simulink model "chap2_6sim"  (Simulink 6.3)
settings: Solver=ode45  StartTime=0.0  StopTime=10  RelTol=1e-3
values from neighbouring files (symbols this model uses):
  K = 1    [chap2_3.m]    (also in chap2_6int.m = 10; chap2_7.m = Kp*tf([1 wi],[1 0]))
  tol = 80    [chap2_3.m]    (also in chap2_6int.m = 1; chap2_9.m)
settings Model: LastModifiedBy=Administrator  ExtModeTrigMode=oneshot  ExtModeArmWhenConnect=off  StrictBusMsg=None
settings DataIOCC: LimitDataPoints=off  SignalLoggingName=sigsOut
settings OptimizationCC: BooleanDataType=off
settings DebuggingCC: SolverPrmCheckMsg=none
settings HardwareCC: TargetUnknown=on

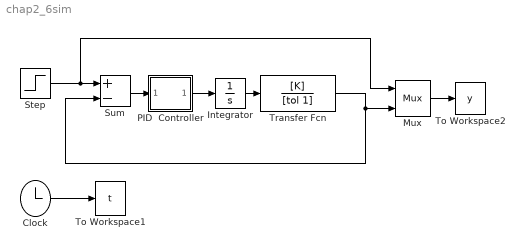
== system chap2_6sim ==
  Clock : Clock
      settings: Decimation=10
  Integrator : Integrator
  Mux : Mux  Inputs=2
  PID  Controller : Subsystem  mask(PID Controller){@1=Kp, @2=0, @3=Kd}
      mask prompts: @1 "Proportional:"; @2 "Integral"; @3 "Derivative:"
      mask help:
      | Enter expressions for proportional, integral, and derivative terms.
      | P+I/s+Ds
      mask init:
      | P=@1; I=@2; D=@3;
      mask Help: This block implements a PID controller where parameters are entered for the Proportional, Integral and Derivative terms. Unmask this block to see how it works. The derivative term is implemented using a true derivative block.
      mask Display: disp('PID')
  Step : Step  Time=0  SampleTime=0
  Sum : Sum  Inputs=+-  SaturateOnIntegerOverflow=on  InputSameDT=on
  To Workspace1 : ToWorkspace  VariableName=t  SampleTime=-1  SaveFormat=Array
  To Workspace2 : ToWorkspace  VariableName=y  SampleTime=-1  SaveFormat=Array
  Transfer Fcn : TransferFcn  Numerator=[K]  Denominator=[tol 1]
  wires:
  Mux/1 -> To Workspace2/1
  Sum/1 -> PID  Controller/1(In_1)
  Transfer Fcn/1 -> Mux/2, Sum/2
  PID  Controller/1(Out_1) -> Integrator/1
  Step/1 -> Mux/1, Sum/1
  Integrator/1 -> Transfer Fcn/1
  Clock/1 -> To Workspace1/1

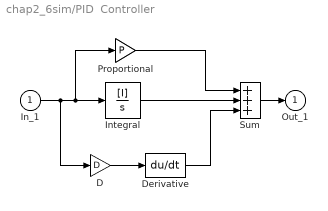
== system chap2_6sim/PID  Controller ==
  In_1 : Inport
  D : Gain  Gain=D  SaturateOnIntegerOverflow=on
  Derivative : Derivative
  Integral : TransferFcn  Numerator=[I]  Denominator=[1 0]
  Proportional : Gain  Gain=P  SaturateOnIntegerOverflow=on
  Sum : Sum  Inputs=+++  SaturateOnIntegerOverflow=on  InputSameDT=on
  Out_1 : Outport  InitialOutput=0
  wires:
  D/1 -> Derivative/1
  Sum/1 -> Out_1/1
  In_1/1 -> D/1, Proportional/1, Integral/1
  Derivative/1 -> Sum/3
  Integral/1 -> Sum/2
  Proportional/1 -> Sum/1
